simulink model "AAAObjectTracking"  (R2023b)
settings: Solver=VariableStepAuto  StartTime=0.0  StopTime=inf  RelTol=1e-3
undefined symbols (not defined in the file): objX, objY, sampleTime
libraries: mobileRoboticsLib x3
settings Model: Creator=gabri  LastModifiedBy=gabri

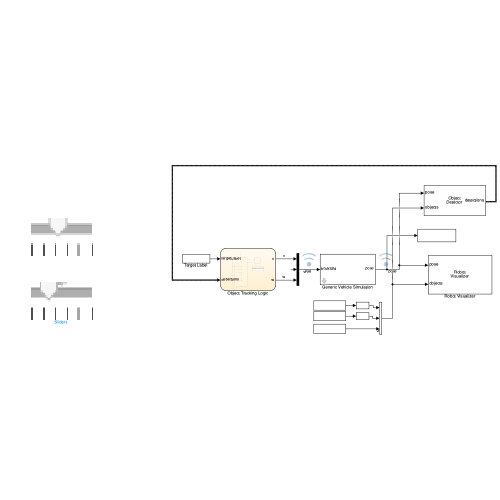
[thumbnail: Simulink's stored preview of the top-level diagram]
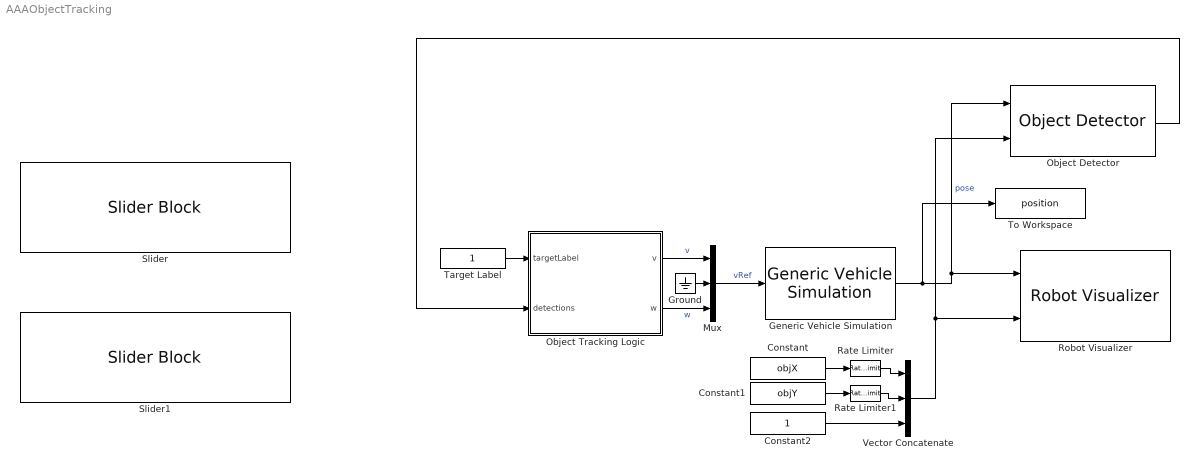
== system AAAObjectTracking ==
  Constant : Constant  Value=objX
  Constant1 : Constant  Value=objY
  Constant2 : Constant
  Generic Vehicle Simulation : mobileRoboticsLib/Utilities/Generic Vehicle Simulation  initX=2  initY=3  initAngle=0  Ts=sampleTime
      settings: SourceProductName=Mobile Robotics Simulation Toolbox
  Ground : Ground
  Mux : Mux  Inputs=3
  Object Detector : mobileRoboticsLib/Environments/Object Detector  sensorOffset=objDetectorOffset  sensorAngle=objDetectorAngle  fieldOfView=objDetectorFOV  maxRange=objDetectorRange  maxDetections=objDetectorMaxHits  sampleTime=-1
      settings: SourceProductName=Mobile Robotics Simulation Toolbox
  Object Tracking Logic : Stateflow chart  TreatAsAtomicUnit=on
  Rate Limiter : RateLimiter  SampleTimeMode=inherited  InitialCondition=objX
  Rate Limiter1 : RateLimiter  SampleTimeMode=inherited  InitialCondition=objX
  Robot Visualizer : mobileRoboticsLib/Environments/Robot Visualizer  Priority=99  robotRadius=0  showTrajectory=on  hasWaypoints=off  hasLidar=off  sensorOffset=[ 0 0 ]  scanAngles=0  hasObjDetector=on  objDetectorOffset=objDetectorOffset  objDetectorAngle=objDetectorAngle  objDetectorFOV=objDetectorFOV  objDetectorMaxRange=objDetectorRange  objectColors=objDetectorColors  objectMarkers=s
  Slider : SliderBlock  ScaleMax=13
  Slider1 : SliderBlock  ScaleMax=13
  Target Label : Constant
  To Workspace : ToWorkspace  VariableName=position  SampleTime=1
  Vector Concatenate : Concatenate  NumInputs=3  Mode=Multidimensional array  ConcatenateDimension=2
  wires:
  Ground/1 -> Mux/2
  Generic Vehicle Simulation/1 -> To Workspace/1, Object Detector/1, Robot Visualizer/1  "pose"
  Vector Concatenate/1 -> Robot Visualizer/2, Object Detector/2
  Object Tracking Logic/2(w) -> Mux/3  "w"
  Mux/1 -> Generic Vehicle Simulation/1  "vRef"
  Object Tracking Logic/1(v) -> Mux/1  "v"
  Object Detector/1 -> Object Tracking Logic/2(detections)
  Target Label/1 -> Object Tracking Logic/1(targetLabel)
  Constant/1 -> Rate Limiter/1
  Rate Limiter1/1 -> Vector Concatenate/2
  Constant1/1 -> Rate Limiter1/1
  Rate Limiter/1 -> Vector Concatenate/1
  Constant2/1 -> Vector Concatenate/3

== stateflow chart AAAObjectTracking/Object Tracking Logic ==
  state TrackObject
    entry, during:
    [range,angle,valid] = findValidObject(targetLabel);
    if valid
    count = 0;
    else
    count = count + 1;
    end
    (default) -> (junction 100)
    TrackObject -> (junction 100) [order 1]
    (junction 100) -> (junction 94) [order 1] : % Set angular speed if
        | % angle outside deadband
        | [abs(angle) > pi/24]
    (junction 100) -> (junction 101) [order 2] : {w = 0;}
    (junction 94) -> (junction 93) : % Proportional
        | % control
        | {w = 1.5*angle;}
    (junction 93) -> (junction 101)
    (junction 101) -> (junction 91)
    (junction 91) -> (junction 90) [order 1] : % Go forward if object is far
        | [range > 1]
    (junction 91) -> (junction 89) [order 2] : {v = 0.1;}
    (junction 90) -> (junction 92) : {v = 0.5;}
    (junction 89) -> (junction 120) [order 2]
    (junction 92) -> (junction 89)
    (junction 89) -> (junction 118) [order 1] : [range < 0.3]{v = 0;}
    (junction 118) -> (junction 125) [order 1] : [abs(angle) > pi/8]
    (junction 125) -> (junction 127) : {w = 0.1 * angle;}
    (junction 118) -> (junction 129) [order 2] : {w = 0.05 * angle;}
    (junction 129) -> (junction 134) [order 2]
    (junction 127) -> (junction 129)
    (junction 129) -> (junction 132) [order 1] : [abs(angle) < 0.02]{w = 0;}
  state SeekObject
    entry:
    v = 0;
    w = 1;
  (default) -> TrackObject : {
      | count = 0;
      | range = 0;
      | angle = 0;
      | }
  TrackObject -> SeekObject [order 1] : [count > 20]
  SeekObject -> TrackObject : [~isempty(detections)]
  data: dist function_output; ang function_output; flag function_output; label function_input; targetLabel input; detections input size=[objDetectorMaxHits,3]; v output; w output; angle local; range local; count local; valid local
  function [dist,ang,flag] = findValidObject(label):
    | function [dist,ang,flag] = findValidObject(label)
    | % Finds the distance (dist) and angle (ang) of the nearest valid
    | % object detected. If an object is found, the (flag) output is true.
    | 
    | % Initialize
    | flag = false;
    | dist = 0;
    | ang = 0;
    | 
    | if ~isempty(detections)
    |     % Loop through all detections
    |     for idx = 1:size(detections,1)
    |         % If a detection matching the target label is found, 
    |         % return it and set the valid flag to true.
    |         if detections(idx,3) == label
    |             dist = detections(idx,1);
    |             ang  = detections(idx,2);
    |             flag = true;
    |             return; 
    |         end
    |     end
    | end
